simulink model "threeDiskOscillatorRig_v2"  (R2024b)
settings: Solver=VariableStepAuto  StartTime=0.0  StopTime=simTime  RelTol=1e-3
values from neighbouring files (symbols this model uses):
  T_s = 4e-3    (= 0.004)    [threeDiskOscillator.m]
libraries: cstblocks x2
settings Model: Creator=nicol  LastModifiedBy=nicol

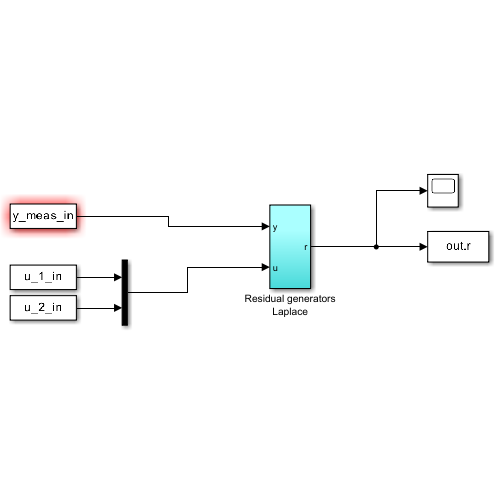
[thumbnail: Simulink's stored preview of the top-level diagram]
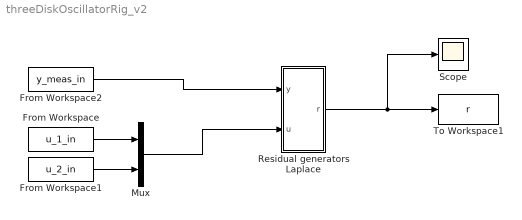
== system threeDiskOscillatorRig_v2 ==
  From Workspace : FromWorkspace  VariableName=u_1_in  SampleTime=T_s
  From Workspace1 : FromWorkspace  VariableName=u_2_in  SampleTime=T_s
  From Workspace2 : FromWorkspace  VariableName=y_meas_in  SampleTime=T_s
  Mux : Mux  Inputs=2
  Residual generators Laplace : Subsystem
  Scope : Scope
  To Workspace1 : ToWorkspace  VariableName=r  SaveFormat=Structure With Time  SampleTime=T_s
  wires:
  From Workspace/1 -> Mux/1
  From Workspace1/1 -> Mux/2
  Mux/1 -> Residual generators Laplace/2(u)
  Residual generators Laplace/1(r) -> To Workspace1/1, Scope/1
  From Workspace2/1 -> Residual generators Laplace/1(y)

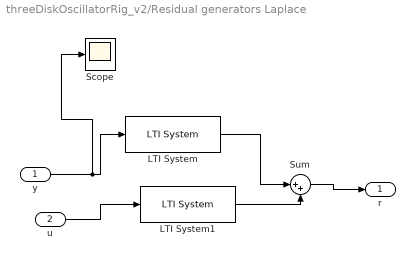
== system threeDiskOscillatorRig_v2/Residual generators Laplace ==
  y : Inport
  u : Inport  Port=2
  LTI System : cstblocks/LTI System  sys=sys_y  IC=[]  PadeOrder=0
  LTI System1 : cstblocks/LTI System  sys=sys_u_normal  IC=[]  PadeOrder=0
  Scope : Scope
  Sum : Sum  Inputs=|++
  r : Outport  VectorParamsAs1DForOutWhenUnconnected=off
  wires:
  Sum/1 -> r/1
  y/1 -> Scope/1, LTI System/1
  u/1 -> LTI System1/1
  LTI System/1 -> Sum/1
  LTI System1/1 -> Sum/2
